simulink model "LQRi_c"  (R2016a)
settings: Solver=VariableStepAuto  StartTime=0.0  StopTime=10.0  RelTol=1e-3
undefined symbols (not defined in the file): LQR_K
settings Model: Creator=mgreiff  LastModifiedBy=mgreiff
settings DataIOCC: LimitDataPoints=on
settings DebuggingCC: AllowSymbolicDim=off
settings ModelReferenceCC: PropagateSignalLabelsOutOfModel=off
settings GRTTargetCC: GeneratePreprocessorConditionals=Use local settings

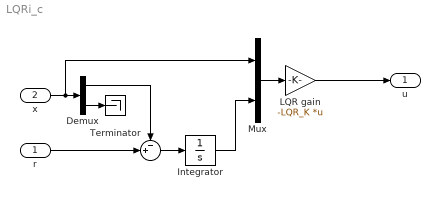
== system LQRi_c ==
  r : Inport  PortDimensions=2
  x : Inport  Port=2  PortDimensions=3
  " " : Sum  Inputs=-+|
  Demux : Demux  Outputs=[2,1]
  Integrator : Integrator
  LQR gain : Gain  Gain=-LQR_K  Multiplication=Matrix(K*u)
  Mux : Mux  Inputs=[3,2]
  Terminator : Terminator
  u : Outport  PortDimensions=1
  wires:
  x/1 -> Mux/1, Demux/1
  Demux/2 -> Terminator/1
  " "/1 -> Integrator/1
  Mux/1 -> LQR gain/1
  LQR gain/1 -> u/1
  r/1 -> " "/2
  Demux/1 -> " "/1
  Integrator/1 -> Mux/2
